simulink model "ciaglu_i_lin"  (R2023a)
settings: Solver=VariableStepAuto  StartTime=0.0  StopTime=200  RelTol=1e-3
values from neighbouring files (symbols this model uses):
  a0 = 0.000531632    [zad1.m]    (also in zad2_8.m; zadanie_dodatkowe.m)
  a1 = 0.0207337    [zad1.m]    (also in zad2_8.m; zadanie_dodatkowe.m)
  a2 = 0.254652    [zad1.m]    (also in zad2_8.m; zadanie_dodatkowe.m)
  alpha1 = -0.3    [zad1.m]    (also in zad2_8.m; zadanie_dodatkowe.m)
  alpha2 = -0.55    [zad1.m]    (also in zad2_8.m; zadanie_dodatkowe.m)
  alpha3 = 0.4    [zad1.m]    (also in zad2_8.m; zadanie_dodatkowe.m)
  alpha4 = 0.21    [zad1.m]    (also in zad2_8.m; zadanie_dodatkowe.m)
  b0 = 0.00122807    [zad1.m]    (also in zad2_8.m; zadanie_dodatkowe.m)
  u0 = 0    [zad2_8.m]    (also in zadanie_dodatkowe.m = 0.5)
settings Model: Creator=adams  LastModifiedBy=adams

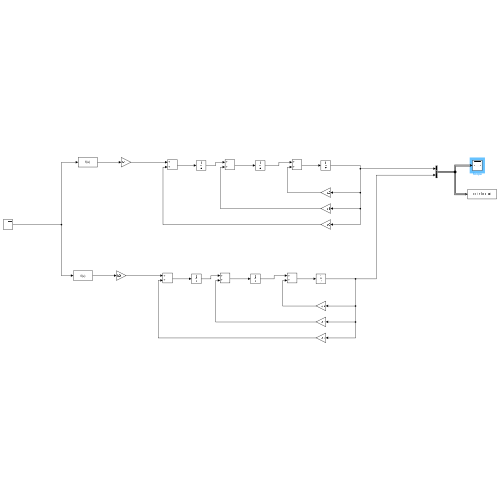
[thumbnail: Simulink's stored preview of the top-level diagram]
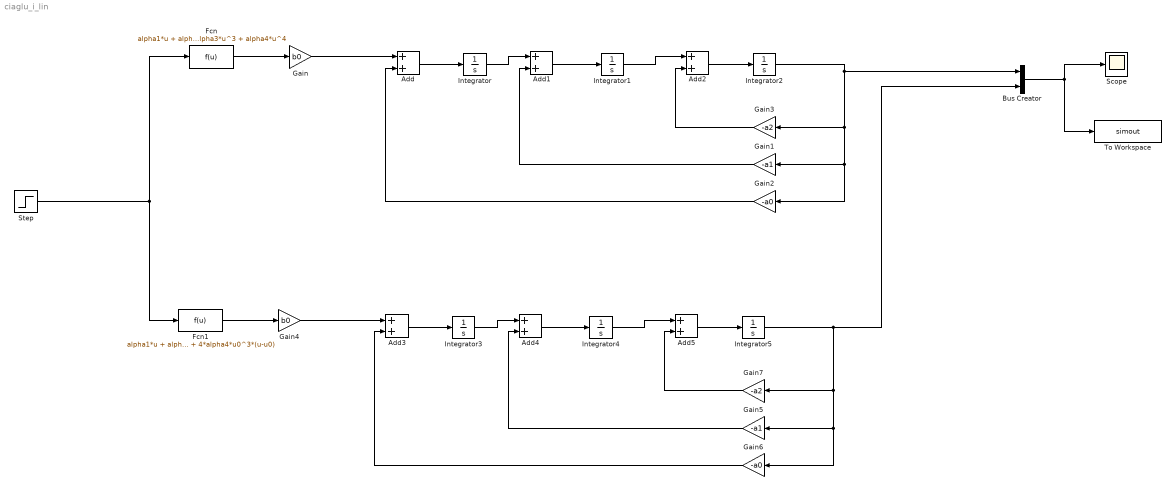
== system ciaglu_i_lin ==
  Add{,1..5} (6 alike) : Sum
  Bus Creator : BusCreator  Inputs=2
  Fcn : Fcn  Expr=alpha1*u + alpha2*u^2 + alpha3*u^3 + alpha4*u^4
  Fcn1 : Fcn  Expr=alpha1*u + alpha2*u0^2+2*alpha2*u0*(u-u0) + alpha3*u0^3 + 3*alpha3*u0^2*(u-u0) + alpha4*u0^4 + 4*alpha4*u0^3*(u-u0)
  Gain : Gain  Gain=b0
  Gain1 : Gain  Gain=-a1
  Gain2 : Gain  Gain=-a0
  Gain3 : Gain  Gain=-a2
  Gain4 : Gain  Gain=b0
  Gain5 : Gain  Gain=-a1
  Gain6 : Gain  Gain=-a0
  Gain7 : Gain  Gain=-a2
  Integrator{,1..5} (6 alike) : Integrator
  Scope : Scope
  Step : Step  After=0.6  SampleTime=0
  To Workspace : ToWorkspace  VariableName=simout  SaveFormat=Timeseries  SampleTime=-1
  wires:
  Step/1 -> Fcn/1, Fcn1/1
  Add2/1 -> Integrator2/1
  Add1/1 -> Integrator1/1
  Integrator2/1 -> Gain2/1, Gain1/1, Gain3/1, Bus Creator/1
  Gain3/1 -> Add2/2
  Integrator1/1 -> Add2/1
  Gain1/1 -> Add1/2
  Integrator/1 -> Add1/1
  Fcn/1 -> Gain/1
  Gain2/1 -> Add/2
  Add/1 -> Integrator/1
  Gain/1 -> Add/1
  Integrator5/1 -> Bus Creator/2, Gain5/1, Gain6/1, Gain7/1
  Fcn1/1 -> Gain4/1
  Gain4/1 -> Add3/1
  Add3/1 -> Integrator3/1
  Add5/1 -> Integrator5/1
  Integrator4/1 -> Add5/1
  Gain7/1 -> Add5/2
  Add4/1 -> Integrator4/1
  Integrator3/1 -> Add4/1
  Gain5/1 -> Add4/2
  Gain6/1 -> Add3/2
  Bus Creator/1 -> Scope/1, To Workspace/1
